simulink model "NMPCLib"  (R2018a)
settings: Solver=VariableStepAuto  StartTime=0.0  StopTime=10.0  RelTol=1e-3  EnableMultiTasking=on
values from neighbouring files (symbols this model uses):
  dU0 = 0*ones(Usize,1)    [go.m]
  U0 = 0*ones(Usize,1)    [go.m]
settings Model: Creator=stajeddi  LastModifiedBy=yesid
settings DataIOCC: LimitDataPoints=on
settings OptimizationCC: LifeSpan=inf
settings DebuggingCC: AllowSymbolicDim=off  SFUnexpectedBacktrackingDiag=warning  SFNoUnconditionalDefaultTransitionDiag=warning  SFExecutionAtInitializationDiag=none
settings ModelReferenceCC: PropagateSignalLabelsOutOfModel=off
settings CodeAppCC: StateflowObjectComments=on
settings GRTTargetCC: TargetLangStandard=C89/C90 (ANSI)
settings ConfigComp: CovMetricSettings=dw  CovHtmlReporting=on  CovSaveCumulativeToWorkspaceVar=on  CovSaveSingleToWorkspaceVar=on  CovExternalEMLEnable=off

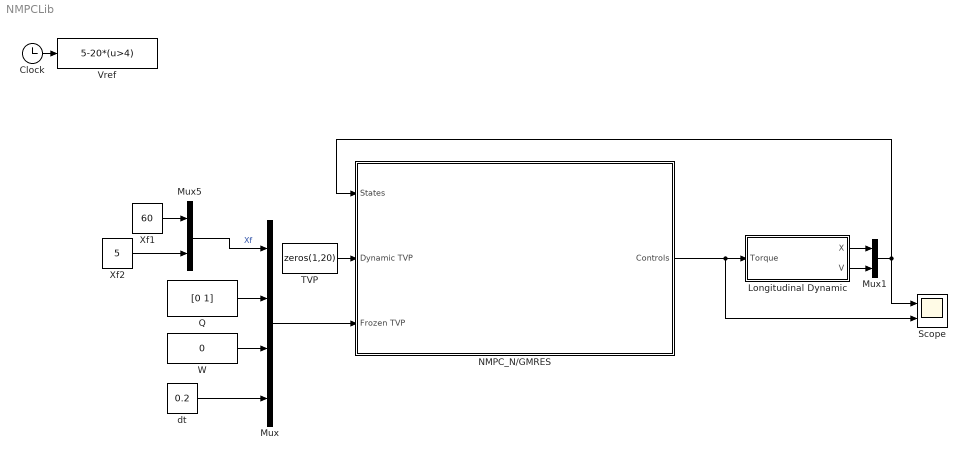
== system NMPCLib ==
  Clock : Clock
  Longitudinal Dynamic : Subsystem
  Mux : Mux
  Mux1 : Mux  Inputs=2
  Mux5 : Mux  Inputs=2
  NMPC_N/GMRES : Subsystem
  Q : Constant  Value=[0 1]
  Scope : Scope  NumInputPorts=2
  TVP : Constant  Value=zeros(1,20)
  Vref : Fcn  Expr=5-20*(u>4)
  W : Constant  Value=0
  Xf1 : Constant  Value=60
  Xf2 : Constant  Value=5
  dt : Constant  Value=0.2
  wires:
  Mux/1 -> NMPC_N/GMRES/3(Frozen TVP)
  Xf1/1 -> Mux5/1
  W/1 -> Mux/3
  dt/1 -> Mux/4
  Mux5/1 -> Mux/1  "Xf"
  Q/1 -> Mux/2
  Longitudinal Dynamic/2(V) -> Mux1/2
  Longitudinal Dynamic/1(X) -> Mux1/1
  Mux1/1 -> Scope/1, NMPC_N/GMRES/1(States)
  NMPC_N/GMRES/1(Controls) -> Scope/2, Longitudinal Dynamic/1(Torque)
  TVP/1 -> NMPC_N/GMRES/2(Dynamic TVP)
  Xf2/1 -> Mux5/2
  Clock/1 -> Vref/1

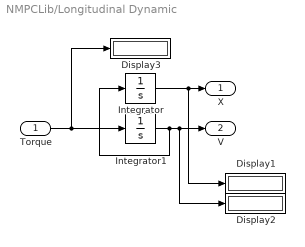
== system NMPCLib/Longitudinal Dynamic ==
  Torque : Inport
  Display1 : Display
  Display2 : Display
  Display3 : Display
  Integrator : Integrator
  Integrator1 : Integrator
  X : Outport
  V : Outport  Port=2
  wires:
  Integrator1/1 -> Integrator/1, Display2/1, V/1
  Torque/1 -> Integrator1/1, Display3/1
  Integrator/1 -> Display1/1, X/1

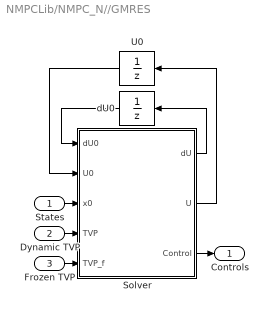
== system NMPCLib/NMPC_N//GMRES ==
  States : Inport
  Dynamic TVP : Inport  Port=2
  Frozen TVP : Inport  Port=3
  Solver : MATLAB Function  TreatAsAtomicUnit=on
  U0 : UnitDelay  InitialCondition=U0  SampleTime=-1
  dU0 : UnitDelay  InitialCondition=dU0  SampleTime=-1
  Controls : Outport
  wires:
  States/1 -> Solver/3(x0)
  Frozen TVP/1 -> Solver/5(TVP_f)
  Solver/3(Control) -> Controls/1
  Solver/2(U) -> U0/1
  U0/1 -> Solver/2(U0)
  Solver/1(dU) -> dU0/1
  dU0/1 -> Solver/1(dU0)
  Dynamic TVP/1 -> Solver/4(TVP)

== matlab function NMPCLib/NMPC_N//GMRES/Solver ==
  data: dU0 input; dU output; U0 input; x0 input; TVP input; U output; Control output; TVP_f input
%% NGMRES  NGMRES NGMRES
function [dU,U,Control] = NMPCBlock(dU0,U0,x0,TVP,TVP_f)
[dU,U,Control]=NMPC(dU0,U0,x0,TVP,TVP_f);
